simulink model "simulink_robo_thiago"  (R2014a)
settings: Solver=ode4  StartTime=0.0  StopTime=Tsim  RelTol=1e-3
values from neighbouring files (symbols this model uses):
  a = 1    [simula_robo_thiago.m]
  b = 0.1    [simula_robo.m]    (also in simula_robo_thiago.m)
  Ic = 1    [simula_robo_thiago.m]
  Kd = 0    [simula_robo.m]    (also in simula_robo_thiago.m)
  Ki = 10.0    (= 10)    [simula_robo.m]    (also in simula_robo_thiago.m = 0)
  Kp = 5.0    (= 5)    [simula_robo.m]    (also in simula_robo_thiago.m = 50)
  m = 100    [simula_robo_thiago.m]
  r = 0.07    [simula_robo.m]    (also in simula_robo_thiago.m)
  thetao = 0.0    (= 0)    [simula_robo.m]    (also in simula_robo_thiago.m)
  Ts = 0.1    [simula_robo.m]    (also in simula_robo_thiago.m)
  xo = 0.0    (= 0)    [simula_robo.m]    (also in simula_robo_thiago.m)
  yo = -0.3    [simula_robo.m]    (also in simula_robo_thiago.m)
libraries: simulink x2
settings Model: Creator=Fabricio  LastModifiedBy=Thiago Lobo
settings DebuggingCC: UnderspecifiedInitializationDetection=Classic  StateNameClashWarn=warning

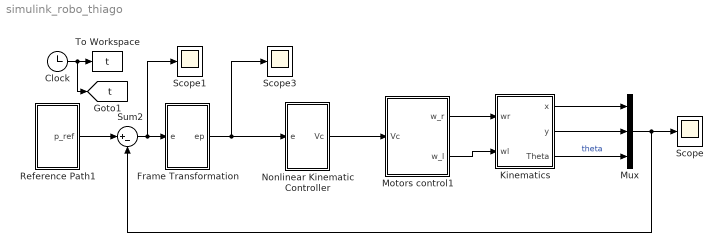
== system simulink_robo_thiago ==
  Clock : Clock
  Frame Transformation : Subsystem
  Kinematics : Subsystem
  Motors control1 : Subsystem
  Mux : Mux  Inputs=3
  Nonlinear Kinematic Controller : Subsystem
  Reference Path1 : Subsystem
  Scope : Scope
      settings: TimeRange=10
  Scope1 : Scope
      settings: TimeRange=10  SaveName=ScopeData2
  Scope3 : Scope
      settings: ShowLegends=on  TimeRange=10  SaveName=ScopeData4
  Sum2 : Sum  Inputs=|+-
  To Workspace : ToWorkspace  VariableName=t  SampleTime=Ts
  tag scope: t=global
  wires:
  Kinematics/2(y) -> Mux/2
  Kinematics/3(Theta) -> Mux/3  "theta"
  Frame Transformation/1(ep) -> Nonlinear Kinematic Controller/1(e), Scope3/1
  Nonlinear Kinematic Controller/1(Vc) -> Motors control1/1(Vc)
  Clock/1 -> [t], To Workspace/1
  Mux/1 -> Sum2/2, Scope/1
  Sum2/1 -> Scope1/1, Frame Transformation/1(e)
  Kinematics/1(x) -> Mux/1
  Reference Path1/1(p_ref) -> Sum2/1
  Motors control1/2(w_l) -> Kinematics/2(wl)
  Motors control1/1(w_r) -> Kinematics/1(wr)

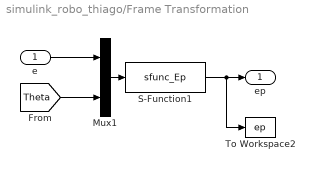
== system simulink_robo_thiago/Frame Transformation ==
  e : Inport
  Mux1 : Mux  Inputs=2
  S-Function1 : S-Function  FunctionName=sfunc_Ep  Parameters=Ts  EnableBusSupport=off
  To Workspace2 : ToWorkspace  VariableName=ep  SampleTime=Ts
  ep : Outport
  wires:
  S-Function1/1 -> To Workspace2/1, ep/1
  Mux1/1 -> S-Function1/1
  e/1 -> Mux1/1
  [Theta] -> Mux1/2

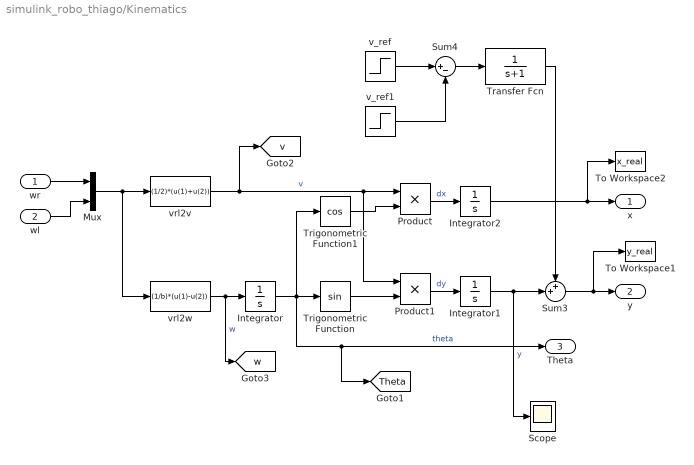
== system simulink_robo_thiago/Kinematics ==
  wr : Inport
  wl : Inport  Port=2
  Integrator : Integrator  InitialCondition=thetao
  Integrator1 : Integrator  InitialCondition=yo
  Integrator2 : Integrator  InitialCondition=xo
  Mux : Mux  Inputs=2
  Product : Product
  Product1 : Product
  Scope : Scope
      settings: TimeRange=10
  Sum3 : Sum  Inputs=++|
  Sum4 : Sum  Inputs=|+-
  To Workspace1 : ToWorkspace  VariableName=y_real  SampleTime=Ts
  To Workspace2 : ToWorkspace  VariableName=x_real  SampleTime=Ts
  Transfer Fcn : TransferFcn  Denominator=[1 1]
  Trigonometric Function : Trigonometry
  Trigonometric Function1 : Trigonometry  Operator=cos
  v_ref : Step  Time=25  After=-0.1  SampleTime=0
  v_ref1 : Step  Time=26  After=-0.1  SampleTime=0
  vrl2v : Fcn  Expr=(1/2)*(u(1)+u(2))
  vrl2w : Fcn  Expr=(1/b)*(u(1)-u(2))
  x : Outport
  y : Outport  Port=2
  Theta : Outport  Port=3
  tag scope: Theta=global, v=global, w=global
  wires:
  wr/1 -> Mux/1
  Trigonometric Function1/1 -> Product/2
  Product/1 -> Integrator2/1  "dx"
  Integrator/1 -> [Theta], Theta/1, Trigonometric Function1/1, Trigonometric Function/1  "theta"
  Integrator1/1 -> Sum3/2, Scope/1  "y"
  Product1/1 -> Integrator1/1  "dy"
  Trigonometric Function/1 -> Product1/2
  Mux/1 -> vrl2w/1, vrl2v/1
  wl/1 -> Mux/2
  vrl2w/1 -> [w], Integrator/1  "w"
  vrl2v/1 -> Product/1, Product1/1, [v]  "v"
  v_ref/1 -> Sum4/1
  v_ref1/1 -> Sum4/2
  Sum4/1 -> Transfer Fcn/1
  Integrator2/1 -> To Workspace2/1, x/1
  Sum3/1 -> To Workspace1/1, y/1
  Transfer Fcn/1 -> Sum3/1

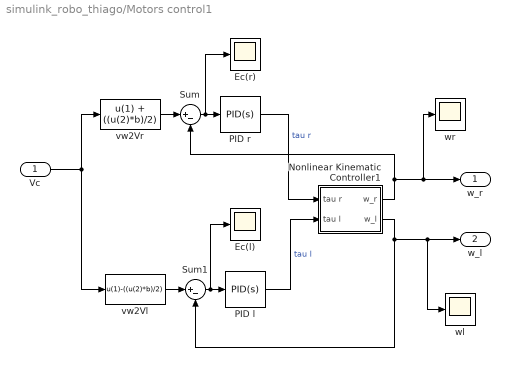
== system simulink_robo_thiago/Motors control1 ==
  Vc : Inport
  Ec(l) : Scope
      settings: SaveName=ScopeData7
  Ec(r) : Scope
      settings: SaveName=ScopeData6
  Nonlinear Kinematic Controller1 : Subsystem
  PID l : simulink/Continuous/PID Controller  Controller=PID  TimeDomain=Continuous-time  SampleTime=1  IntegratorMethod=Forward Euler  FilterMethod=Forward Euler  Form=Parallel  P=Kp  I=Ki  D=Kd  N=100  InitialConditionSource=internal  InitialConditionForIntegrator=0  InitialConditionForFilter=0  ExternalReset=none  LimitOutput=off  UpperSaturationLimit=inf  LowerSaturationLimit=-inf  LinearizeAsGain=on  AntiWindupMode=none  Kb=1  TrackingMode=off  Kt=1  PParamMin=[]  PParamMax=[]  IParamMin=[]  IParamMax=[]  DParamMin=[]  DParamMax=[]  NParamMin=[]  NParamMax=[]  KbParamMin=[]  KbParamMax=[]  KtParamMin=[]  KtParamMax=[]  POutMin=[]  POutMax=[]  IOutMin=[]  IOutMax=[]  DOutMin=[]  DOutMax=[]  NOutMin=[]  NOutMax=[]  KbOutMin=[]  KbOutMax=[]  KtOutMin=[]  KtOutMax=[]  IntegratorOutMin=[]  IntegratorOutMax=[]  FilterOutMin=[]  FilterOutMax=[]  SumOutMin=[]  SumOutMax=[]  SumI1OutMin=[]  SumI1OutMax=[]  SumI2OutMin=[]  SumI2OutMax=[]  SumI3OutMin=[]  SumI3OutMax=[]  SumDOutMin=[]  SumDOutMax=[]  SaturationOutMin=[]  SaturationOutMax=[]  IntegratorContinuousStateAttributes=''  IntegratorStateMustResolveToSignalObject=off  IntegratorRTWStateStorageClass=Auto  FilterContinuousStateAttributes=''  FilterStateMustResolveToSignalObject=off  FilterRTWStateStorageClass=Auto
  PID r : simulink/Continuous/PID Controller  Controller=PID  TimeDomain=Continuous-time  SampleTime=1  IntegratorMethod=Forward Euler  FilterMethod=Forward Euler  Form=Parallel  P=Kp  I=Ki  D=Kd  N=100  InitialConditionSource=internal  InitialConditionForIntegrator=0  InitialConditionForFilter=0  ExternalReset=none  LimitOutput=off  UpperSaturationLimit=inf  LowerSaturationLimit=-inf  LinearizeAsGain=on  AntiWindupMode=none  Kb=1  TrackingMode=off  Kt=1  PParamMin=[]  PParamMax=[]  IParamMin=[]  IParamMax=[]  DParamMin=[]  DParamMax=[]  NParamMin=[]  NParamMax=[]  KbParamMin=[]  KbParamMax=[]  KtParamMin=[]  KtParamMax=[]  POutMin=[]  POutMax=[]  IOutMin=[]  IOutMax=[]  DOutMin=[]  DOutMax=[]  NOutMin=[]  NOutMax=[]  KbOutMin=[]  KbOutMax=[]  KtOutMin=[]  KtOutMax=[]  IntegratorOutMin=[]  IntegratorOutMax=[]  FilterOutMin=[]  FilterOutMax=[]  SumOutMin=[]  SumOutMax=[]  SumI1OutMin=[]  SumI1OutMax=[]  SumI2OutMin=[]  SumI2OutMax=[]  SumI3OutMin=[]  SumI3OutMax=[]  SumDOutMin=[]  SumDOutMax=[]  SaturationOutMin=[]  SaturationOutMax=[]  IntegratorContinuousStateAttributes=''  IntegratorStateMustResolveToSignalObject=off  IntegratorRTWStateStorageClass=Auto  FilterContinuousStateAttributes=''  FilterStateMustResolveToSignalObject=off  FilterRTWStateStorageClass=Auto
  Sum : Sum  Inputs=|+-
  Sum1 : Sum  Inputs=|+-
  vw2Vl : Fcn  Expr=u(1)-((u(2)*b)/2)
  vw2Vr : Fcn  Expr=u(1) + ((u(2)*b)/2)
  wl : Scope
      settings: SaveName=ScopeData5
  wr : Scope
      settings: SaveName=ScopeData3
  w_r : Outport
  w_l : Outport  Port=2
  wires:
  Vc/1 -> vw2Vr/1, vw2Vl/1
  PID r/1 -> Nonlinear Kinematic Controller1/1(tau r)  "tau r"
  Sum/1 -> Ec(r)/1, PID r/1
  PID l/1 -> Nonlinear Kinematic Controller1/2(tau l)  "tau l"
  vw2Vl/1 -> Sum1/1
  Sum1/1 -> Ec(l)/1, PID l/1
  Nonlinear Kinematic Controller1/1(w_r) -> wr/1, w_r/1, Sum/2
  Nonlinear Kinematic Controller1/2(w_l) -> wl/1, w_l/1, Sum1/2
  vw2Vr/1 -> Sum/1

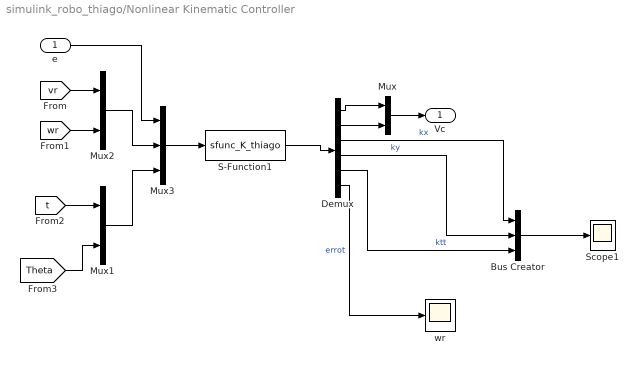
== system simulink_robo_thiago/Nonlinear Kinematic Controller ==
  e : Inport
  Bus Creator : BusCreator  Inputs=3
  Demux : Demux  Outputs=6
  Mux : Mux  Inputs=2
  Mux1 : Mux  Inputs=2
  Mux2 : Mux  Inputs=2
  Mux3 : Mux  Inputs=3
  S-Function1 : S-Function  FunctionName=sfunc_K_thiago  Parameters=Ts  EnableBusSupport=off
  Scope1 : Scope
      settings: ShowLegends=on  TimeRange=10  SaveName=ScopeData8
  wr : Scope
      settings: SaveName=ScopeData9
  Vc : Outport
  wires:
  [Theta] -> Mux1/2
  [t] -> Mux1/1
  Mux3/1 -> S-Function1/1
  [vr] -> Mux2/1
  [wr] -> Mux2/2
  Mux2/1 -> Mux3/2
  Mux1/1 -> Mux3/3
  e/1 -> Mux3/1
  S-Function1/1 -> Demux/1
  Demux/5 -> Bus Creator/3  "ktt"
  Demux/4 -> Bus Creator/2  "ky"
  Demux/3 -> Bus Creator/1  "kx"
  Demux/2 -> Mux/2
  Demux/1 -> Mux/1
  Mux/1 -> Vc/1
  Bus Creator/1 -> Scope1/1
  Demux/6 -> wr/1  "errot"

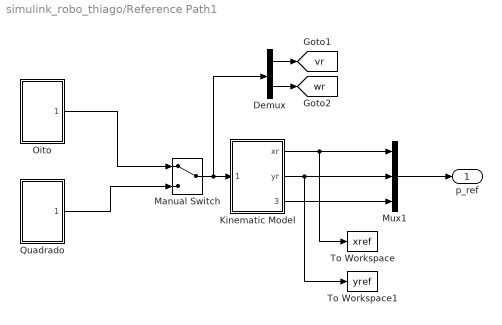
== system simulink_robo_thiago/Reference Path1 ==
  Demux : Demux  Outputs=2
  Kinematic Model : Subsystem
  Manual Switch : ManualSwitch
  Mux1 : Mux  Inputs=3
  Oito : Subsystem
  Quadrado : Subsystem
  To Workspace : ToWorkspace  VariableName=xref  SampleTime=Ts
  To Workspace1 : ToWorkspace  VariableName=yref  SampleTime=Ts
  p_ref : Outport
  tag scope: vr=global, wr=global
  wires:
  Kinematic Model/1(xr) -> To Workspace/1, Mux1/1
  Kinematic Model/3(thetar) -> Mux1/3
  Mux1/1 -> p_ref/1
  Kinematic Model/2(yr) -> To Workspace1/1, Mux1/2
  Oito/1(vw_ref) -> Manual Switch/1
  Quadrado/1(vw_ref) -> Manual Switch/2
  Demux/1 -> [vr]
  Demux/2 -> [wr]
  Manual Switch/1 -> Demux/1, Kinematic Model/1(vw_ref)

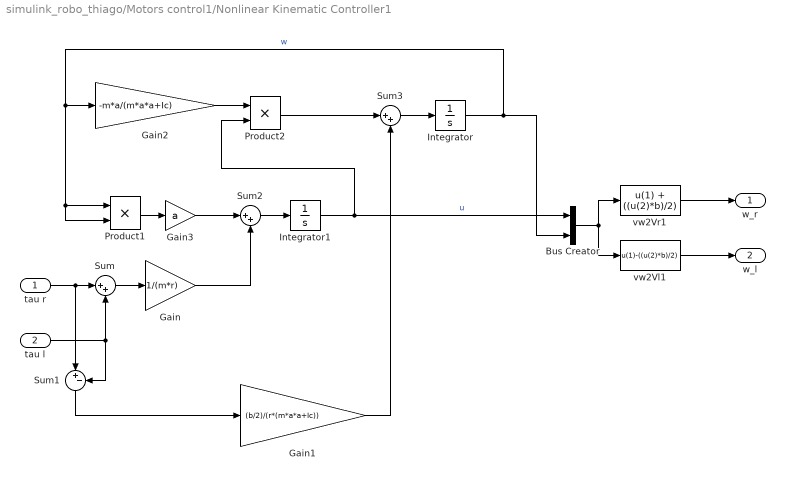
== system simulink_robo_thiago/Motors control1/Nonlinear Kinematic Controller1 ==
  tau r : Inport
  tau l : Inport  Port=2
  Bus Creator : BusCreator  Inputs=2
  Gain : Gain  Gain=1/(m*r)
  Gain1 : Gain  Gain=(b/2)/(r*(m*a*a+Ic))
  Gain2 : Gain  Gain=-m*a/(m*a*a+Ic)
  Gain3 : Gain  Gain=a
  Integrator : Integrator
  Integrator1 : Integrator
  Product1 : Product
  Product2 : Product
  Sum : Sum  Inputs=|++
  Sum1 : Sum  Inputs=|+-
  Sum2 : Sum  Inputs=|++
  Sum3 : Sum  Inputs=|++
  vw2Vl1 : Fcn  Expr=u(1)-((u(2)*b)/2)
  vw2Vr1 : Fcn  Expr=u(1) + ((u(2)*b)/2)
  w_r : Outport
  w_l : Outport  Port=2
  wires:
  tau r/1 -> Sum1/1, Sum/1
  tau l/1 -> Sum/2, Sum1/2
  Sum/1 -> Gain/1
  Product1/1 -> Gain3/1
  Gain3/1 -> Sum2/1
  Gain/1 -> Sum2/2
  Sum1/1 -> Gain1/1
  Product2/1 -> Sum3/1
  Gain1/1 -> Sum3/2
  Integrator1/1 -> Product2/2, Bus Creator/1  "u"
  Sum2/1 -> Integrator1/1
  Sum3/1 -> Integrator/1
  Integrator/1 -> Gain2/1, Product1/1, Product1/2, Bus Creator/2  "w"
  vw2Vr1/1 -> w_r/1
  vw2Vl1/1 -> w_l/1
  Bus Creator/1 -> vw2Vl1/1, vw2Vr1/1
  Gain2/1 -> Product2/1

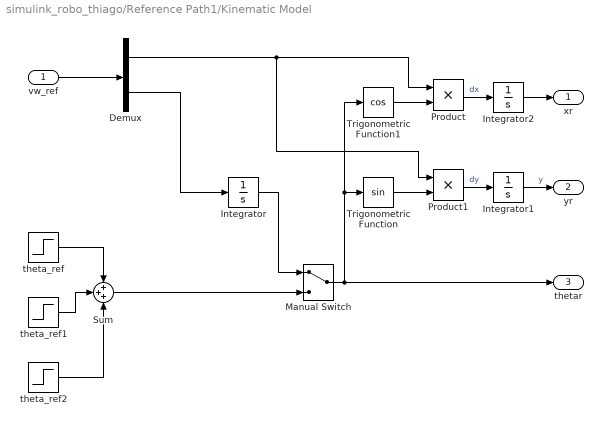
== system simulink_robo_thiago/Reference Path1/Kinematic Model ==
  vw_ref : Inport
  Demux : Demux  Outputs=2
  Integrator : Integrator
  Integrator1 : Integrator
  Integrator2 : Integrator
  Manual Switch : ManualSwitch
  Product : Product
  Product1 : Product
  Sum : Sum  Inputs=+++
  Trigonometric Function : Trigonometry
  Trigonometric Function1 : Trigonometry  Operator=cos
  theta_ref : Step  Time=20  After=pi/2  SampleTime=0
  theta_ref1 : Step  Time=40  After=pi/2  SampleTime=0
  theta_ref2 : Step  Time=60  After=pi/2  SampleTime=0
  xr : Outport
  yr : Outport  Port=2
  thetar : Outport  Port=3
  wires:
  Trigonometric Function1/1 -> Product/2
  Product/1 -> Integrator2/1  "dx"
  Integrator/1 -> Manual Switch/1
  Integrator1/1 -> yr/1  "y"
  Product1/1 -> Integrator1/1  "dy"
  Integrator2/1 -> xr/1
  Trigonometric Function/1 -> Product1/2
  Demux/1 -> Product/1, Product1/1
  Demux/2 -> Integrator/1
  vw_ref/1 -> Demux/1
  theta_ref/1 -> Sum/1
  theta_ref1/1 -> Sum/2
  theta_ref2/1 -> Sum/3
  Sum/1 -> Manual Switch/2
  Manual Switch/1 -> Trigonometric Function1/1, Trigonometric Function/1, thetar/1

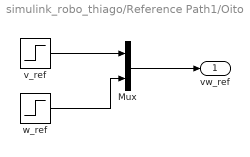
== system simulink_robo_thiago/Reference Path1/Oito ==
  Mux : Mux  Inputs=2
  v_ref : Step  Before=10  After=10  SampleTime=0
  w_ref : Step  Time=18  Before=0.35  After=-0.35  SampleTime=0
  vw_ref : Outport
  wires:
  v_ref/1 -> Mux/1
  w_ref/1 -> Mux/2
  Mux/1 -> vw_ref/1

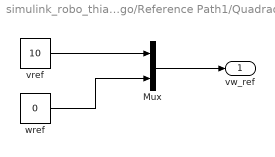
== system simulink_robo_thiago/Reference Path1/Quadrado ==
  Mux : Mux  Inputs=2
  vref : Constant  Value=10
  wref : Constant  Value=0
  vw_ref : Outport
  wires:
  vref/1 -> Mux/1
  wref/1 -> Mux/2
  Mux/1 -> vw_ref/1
